simulink library "INT_GlbDa_LSum"  (R2016b)
settings: Solver=VariableStepAuto  StartTime=0.0  StopTime=10.0  RelTol=1e-3
settings Model: Creator=liutao  LastModifiedBy=liutao

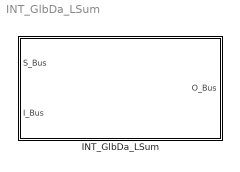
== system INT_GlbDa_LSum ==
  INT_GlbDa_LSum : Subsystem

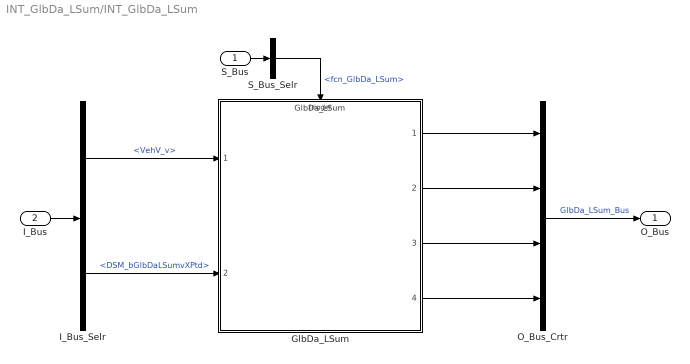
== system INT_GlbDa_LSum/INT_GlbDa_LSum ==
  S_Bus : Inport
  I_Bus : Inport  Port=2
  GlbDa_LSum : ModelReference  ModelNameDialog=GlbDa_LSum  SimulationMode=Normal  ModelReferenceVersion=1.22  TriggerPortName=function  TriggerPortTriggerType=function-call  TriggerPortStatesWhenEnabling=held
  I_Bus_Selr : BusSelector  OutputSignals=VehV_v,DSM_bGlbDaLSumvXPtd
  O_Bus_Crtr : BusCreator  Inputs=4
  S_Bus_Selr : BusSelector  OutputSignals=fcn_GlbDa_LSum
  O_Bus : Outport
  wires:
  S_Bus_Selr/1 -> GlbDa_LSum/Trigger  "<fcn_GlbDa_LSum>"
  S_Bus/1 -> S_Bus_Selr/1
  I_Bus/1 -> I_Bus_Selr/1
  I_Bus_Selr/1 -> GlbDa_LSum/1  "<VehV_v>"
  I_Bus_Selr/2 -> GlbDa_LSum/2  "<DSM_bGlbDaLSumvXPtd>"
  O_Bus_Crtr/1 -> O_Bus/1  "GlbDa_LSum_Bus"
  GlbDa_LSum/1 -> O_Bus_Crtr/1
  GlbDa_LSum/2 -> O_Bus_Crtr/2
  GlbDa_LSum/3 -> O_Bus_Crtr/3
  GlbDa_LSum/4 -> O_Bus_Crtr/4
